simulink model "pendule_inv_etu"  (R2022a)
settings: Solver=VariableStepAuto  StartTime=0.0  StopTime=10.0  RelTol=1e-3
values from neighbouring files (symbols this model uses):
  g = 9.81    [simu_pendule_inv_capteur_etu.m]
  K = [10 1]    [simu_pendule_inv_capteur_etu.m]
  l = 10    [simu_pendule_inv_capteur_etu.m]
  ue = 0    [simu_pendule_inv_capteur_etu.m]
  xe = [0 0]'    [simu_pendule_inv_capteur_etu.m]
undefined symbols (not defined in the file or in its folder): x0
settings Model: Creator=melallem  LastModifiedBy=elgue
settings DebuggingCC: UnconnectedInputMsg=warning  UnconnectedOutputMsg=warning  UnconnectedLineMsg=warning
settings RTWCC: DLArmComputeVersion=19.05

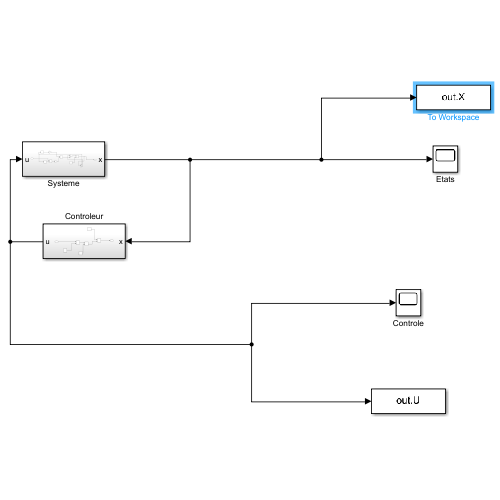
[thumbnail: Simulink's stored preview of the top-level diagram]
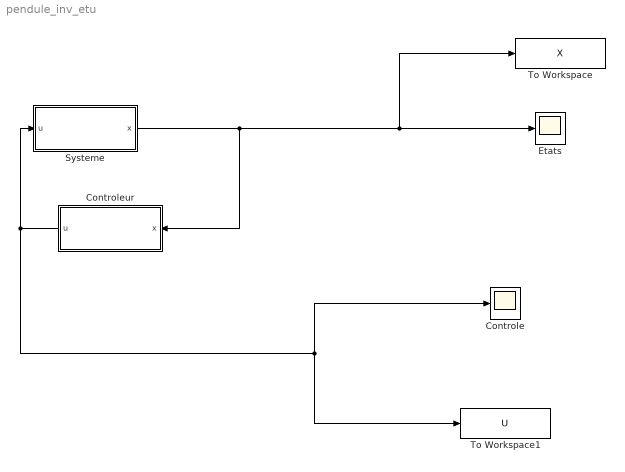
== system pendule_inv_etu ==
  Controle : Scope
  Controleur : Subsystem
  Etats : Scope
  Systeme : Subsystem
  To Workspace : ToWorkspace  VariableName=X  SaveFormat=Timeseries  SampleTime=-1
  To Workspace1 : ToWorkspace  VariableName=U  SaveFormat=Timeseries  SampleTime=-1
  wires:
  Systeme/1(x) -> To Workspace/1, Etats/1, Controleur/1(x)
  Controleur/1(u) -> To Workspace1/1, Controle/1, Systeme/1(u)

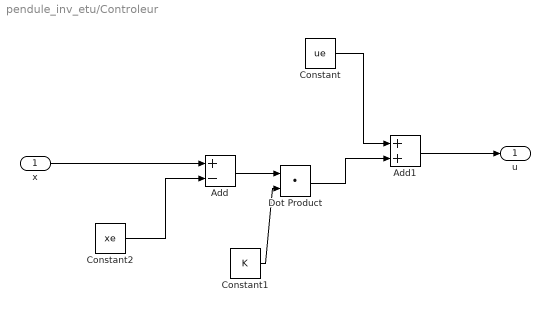
== system pendule_inv_etu/Controleur ==
  x : Inport
  Add : Sum  Inputs=+-
  Add1 : Sum
  Constant : Constant  Value=ue
  Constant1 : Constant  Value=K
  Constant2 : Constant  Value=xe
  Dot Product : DotProduct  OutDataTypeStr=Inherit: Inherit via internal rule
  u : Outport
  wires:
  x/1 -> Add/1
  Add/1 -> Dot Product/1
  Dot Product/1 -> Add1/2
  Add1/1 -> u/1
  Constant2/1 -> Add/2
  Constant1/1 -> Dot Product/2
  Constant/1 -> Add1/1

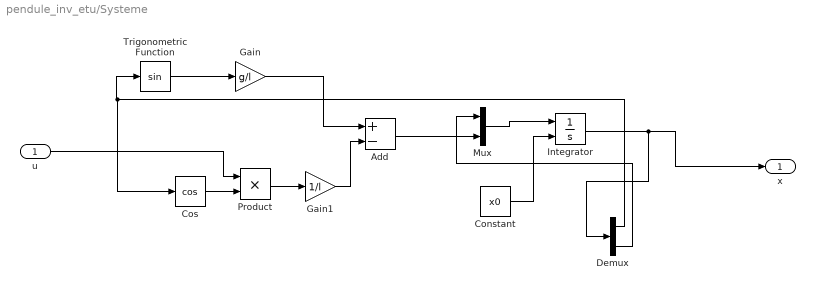
== system pendule_inv_etu/Systeme ==
  u : Inport
  Add : Sum  Inputs=+-
  Constant : Constant  Value=x0
  Cos : Trigonometry  Operator=cos
  Demux : Demux  Outputs=2
  Gain : Gain  Gain=g/l
  Gain1 : Gain  Gain=1/l
  Integrator : Integrator  InitialConditionSource=external
  Mux : Mux  Inputs=2
  Product : Product
  Trigonometric Function : Trigonometry
  x : Outport
  wires:
  u/1 -> Product/1
  Cos/1 -> Product/2
  Constant/1 -> Integrator/2
  Mux/1 -> Integrator/1
  Integrator/1 -> Demux/1, x/1
  Demux/2 -> Mux/1
  Add/1 -> Mux/2
  Trigonometric Function/1 -> Gain/1
  Gain/1 -> Add/1
  Gain1/1 -> Add/2
  Product/1 -> Gain1/1
  Demux/1 -> Cos/1, Trigonometric Function/1
